simulink model "Drive"  (R2018b)
settings: Solver=VariableStepAuto  StartTime=0.0  StopTime=10.0  RelTol=1e-3
settings Model: Creator=kekos  LastModifiedBy=kekos

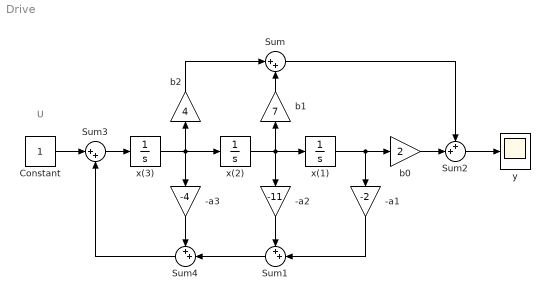
== system Drive ==
  note: U
  -a1 : Gain  Gain=-2
  -a2 : Gain  Gain=-11
  -a3 : Gain  Gain=-4
  Constant : Constant
  Sum : Sum  Inputs=|++
  Sum1 : Sum  Inputs=++|
  Sum2 : Sum  Inputs=++|
  Sum3 : Sum  Inputs=|++
  Sum4 : Sum  Inputs=++|
  b0 : Gain  Gain=2
  b1 : Gain  Gain=7
  b2 : Gain  Gain=4
  x(1) : Integrator  InitialCondition=3.4
  x(2) : Integrator  InitialCondition=3.4
  x(3) : Integrator  InitialCondition=3.4
  y : Scope
  wires:
  x(3)/1 -> -a3/1, b2/1, x(2)/1
  x(2)/1 -> -a2/1, x(1)/1, b1/1
  x(1)/1 -> b0/1, -a1/1
  b1/1 -> Sum/2
  -a2/1 -> Sum1/1
  b0/1 -> Sum2/2
  Sum/1 -> Sum2/1
  b2/1 -> Sum/1
  Constant/1 -> Sum3/1
  Sum3/1 -> x(3)/1
  -a1/1 -> Sum1/2
  Sum1/1 -> Sum4/2
  -a3/1 -> Sum4/1
  Sum4/1 -> Sum3/2
  Sum2/1 -> y/1
